simulink model "motor_response_sim"  (R2021a)
settings: Solver=VariableStepAuto  StartTime=0.0  StopTime=0.07  RelTol=1e-3
undefined symbols (not defined in the file): c, I, Kb, KT, La, Ra
settings Model: Creator=spbro  LastModifiedBy=spbro

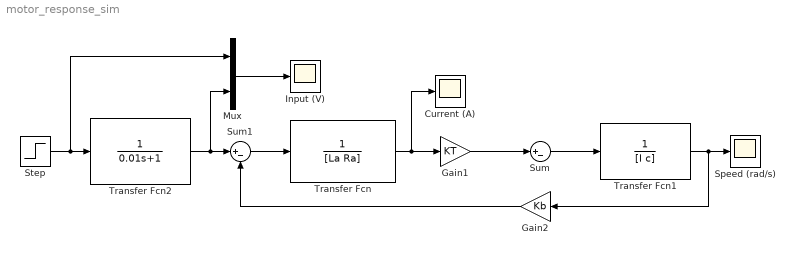
== system motor_response_sim ==
  Current (A) : Scope
  Gain1 : Gain  Gain=KT
  Gain2 : Gain  Gain=Kb
  Input (V) : Scope
  Mux : Mux  Inputs=2
  Speed (rad/s) : Scope
  Step : Step  Time=0  After=10  SampleTime=0
  Sum : Sum  Inputs=|+-
  Sum1 : Sum  Inputs=|+-
  Transfer Fcn : TransferFcn  Denominator=[La Ra]
  Transfer Fcn1 : TransferFcn  Denominator=[I c]
  Transfer Fcn2 : TransferFcn  Denominator=[0.01 1]
  wires:
  Transfer Fcn1/1 -> Gain2/1, Speed (rad/s)/1
  Transfer Fcn2/1 -> Sum1/1, Mux/2
  Mux/1 -> Input (V)/1
  Gain1/1 -> Sum/1
  Gain2/1 -> Sum1/2
  Sum1/1 -> Transfer Fcn/1
  Sum/1 -> Transfer Fcn1/1
  Transfer Fcn/1 -> Gain1/1, Current (A)/1
  Step/1 -> Transfer Fcn2/1, Mux/1
